simulink model "zad3model"  (R2012b)
settings: Solver=ode45  StartTime=0.0  StopTime=10.0  RelTol=1e-3
libraries: simulink x1
settings Model: Creator=VoAnder  LastModifiedBy=VoAnder

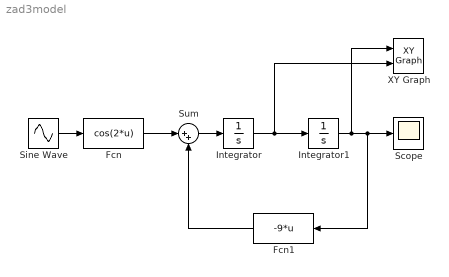
== system zad3model ==
  Fcn : Fcn  Expr=cos(2*u)
  Fcn1 : Fcn  Expr=-9*u
  Integrator : Integrator
  Integrator1 : Integrator
  Scope : Scope
  Sine Wave : Sin  SampleTime=0
  Sum : Sum  Inputs=|++
  XY Graph : simulink/Sinks/XY Graph  xmin=-1  xmax=1  ymin=-1  ymax=1  st=-1
  wires:
  Sine Wave/1 -> Fcn/1
  Fcn/1 -> Sum/1
  Integrator/1 -> XY Graph/2, Integrator1/1
  Integrator1/1 -> XY Graph/1, Fcn1/1, Scope/1
  Fcn1/1 -> Sum/2
  Sum/1 -> Integrator/1
